simulink model "ControlModel"  (R2020b)
settings: Solver=VariableStepAuto  StartTime=0.0  StopTime=3  FixedStep=0.00001  RelTol=1e-3
InitFcn:
  | s = tf('s');
  | Telec = 1/10000000;
  | Tmech = Telec * 10;
  | CW = 1;
  | CCW = -1;
undefined symbols (not defined in the file or in its folder): DiscIntNeverNeededParam, lag, lead, magnitude, notch, rad
libraries: cstblocks x41, sharedtransform x7, simulink x6, aerolibutil x4, aerolibconvert2 x4, simulink_extras x3, sharedutil x1
(part 1 of 2)
settings Model: Creator=Iftah  LastModifiedBy=vguidance01

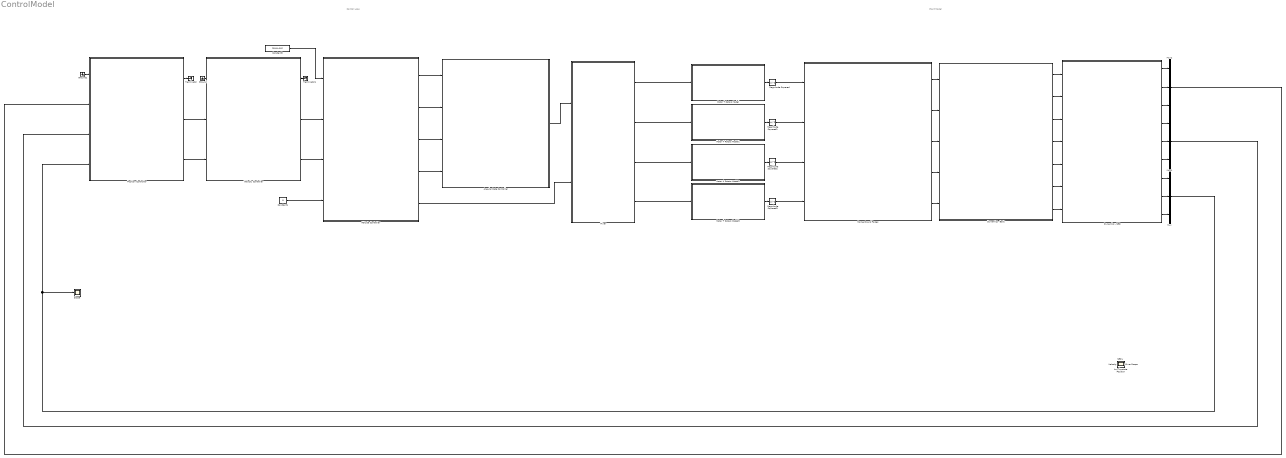
== system ControlModel ==
  note: Plant Model
  note: Control Loop
  Angular Rate Controller : Subsystem  mask{MC_ROLLRATE_K=1, MC_ROLLRATE_P=3, MC_ROLLRATE_I=0.8, MC_ROLLRATE_D=0.4, MC_RR_INT_LIM=101, MC_PITCHRATE_K=1, MC_PITCHRATE_P=3, MC_PITCHRATE_I=0.6, MC_PITCHRATE_D=0.4, MC_PR_INT_LIM=100, MC_YAWRATE_K=1, MC_YAWRATE_P=0.2, MC_YAWRATE_I=0.08, MC_YAWRATE_D=0.001, MC_YR_INT_LIM=100, IMU_DGYRO_CUTOFF=0, IMU_GYRO_CUTOFF=0}
      mask prompts: MC_ROLLRATE_K "MC_ROLLRATE_K ="; MC_ROLLRATE_P "MC_ROLLRATE_P ="; MC_ROLLRATE_I "MC_ROLLRATE_I ="; MC_ROLLRATE_D "MC_ROLLRATE_D ="; MC_RR_INT_LIM "MC_RR_INT_LIM ="; MC_PITCHRATE_K "MC_PITCHRATE_K ="; MC_PITCHRATE_P "MC_PITCHRATE_P ="; MC_PITCHRATE_I "MC_PITCHRATE_I ="; MC_PITCHRATE_D "MC_PITCHRATE_D ="; MC_PR_INT_LIM "MC_PR_INT_LIM ="; MC_YAWRATE_K "MC_YAWRATE_K ="; MC_YAWRATE_P "MC_YAWRATE_P ="; MC_YAWRATE_I "MC_YAWRATE_I ="; MC_YAWRATE_D "MC_YAWRATE_D ="; MC_YR_INT_LIM "MC_YR_INT_LIM ="; IMU_DGYRO_CUTOFF "IMU_DGYRO_CUTOFF ="; IMU_GYRO_CUTOFF "IMU_GYRO_CUTOFF ="
      mask DialogControl DescTextVar Prompt: Angular rate controller, based on PX4 architecture
      mask DialogControl ROLL Prompt: Roll
      mask DialogControl PITCH Prompt: Pitch
      mask DialogControl YAW Prompt: Yaw
      mask Display:
      | disp('Angular Rate Controller')
      | 
      | port_label('input',1,'d\phi_{cmd}','texmode','on')
      | port_label('input',2,'d\theta_{cmd}','texmode','on')
      | port_label('input',3,'d\psi_{cmd}','texmode','on')
      | port_label('input',4,'Gyro','texmode','on')
      | 
      | port_label('output',1,'\delta_{cmd}','texmode','on')
  Attitude Controller : Subsystem  mask{MC_ROLL_P=1, MC_ROLLRATE_MAX=0.5, MC_ACRO_R_MAX=10, MC_YAW_WEIGHT=0.1, m=1.37}
      mask prompts: MC_ROLL_P "MC_ROLL_P ="; MC_ROLLRATE_MAX "MC_ROLLRATE_MAX ="; MC_ACRO_R_MAX "MC_ACRO_R_MAX ="; MC_YAW_WEIGHT "MC_YAW_WEIGHT ="; m "m [kg] ="
      mask DialogControl DescTextVar Prompt: Attitude Controller - based on PX4 architecture
      mask Display:
      | disp('Attitude Controller')
      | 
      | port_label('input',1,'ACCEL. S.P')
      | port_label('input',3,'Accel')
      | port_label('input',2,'Gyro')
      | port_label('input',4,'\psi_{cmd}','texmode','on')
      | 
      | port_label('output',1,'d\phi_{cmd}','texmode','on')
      | port_label('output',2,'d\theta_{cmd}','texmode','on')
      | port_label('output',3,'d\psi_{cmd}','texmode','on')
      | port_label('output',4,'Gyro','texmode','on')
      | port_label('output',5,'Thrust_{cmd}','texmode','on')
  Constant1 : Constant  Value=0  SampleTime=Tmech
  Constant3 : Constant  Value=[10;0;-10]  SampleTime=Tmech
  Dynamics - Body : Subsystem  mask{Ixx=0.0115118, Iyy=0.0365651, Izz=0.0290742, Jr=2.8e-6, d=0.25}
      mask prompts: Ixx "Ixx [kg*m^2] ="; Iyy "Iyy [kg*m^2] ="; Izz "Izz [kg*m^2]="; Jr "Jl [kg*m^2]="; d "d [m] ="
      mask DialogControl DescTextVar Prompt: This model represents the body-frame dyanmics. Enter the MOIs of the system
      mask Display:
      | disp('Body Dyanmics','texmode','on')
      | 
      | port_label('input',1,'T','texmode','on')
      | port_label('input',2,'Roll Thrust','texmode','on')
      | port_label('input',3,'Pitch Thrust','texmode','on')
      | port_label('input',4,'Yaw Thrust','texmode','on')
      | port_label('input',5,'Angular Velocity','texmode','on')
      | 
      | port_label('output',2,'\phi','texmode','on')
      | port_label('output',3,'\theta','texmode','on')
      | port_label('output',4,'\psi','texmode','on')
      | port_label('output',1,'T','texmode','on')
      | port_label('output',5,'d\phi','texmode','on')
      | port_label('output',6,'d\theta','texmode','on')
      | port_label('output',7,'d\psi','texmode','on')
  Dynamics - NED : Subsystem  mask{g=9.81, m=1.37, Ax=0.007, Ay=0.007, Az=0.007}
      mask prompts: g "g [m/s^2] ="; m "m [kg] ="; Ax "Ax [kg/s] ="; Ay "Ay [kg/s]="; Az "Az [kg/s]="
      mask DialogControl DescTextVar Prompt: This block transform the body dyanmics to NED. Choose the mass, gravity, and Ax,Ay,Az - drag coeff.
      mask Display:
      | disp('NED Dyanmics','texmode','on')
      | 
      | port_label('input',2,'\phi','texmode','on')
      | port_label('input',3,'\theta','texmode','on')
      | port_label('input',4,'\psi','texmode','on')
      | port_label('input',1,'T','texmode','on')
      | port_label('input',5,'d\phi','texmode','on')
      | port_label('input',6,'d\theta','texmode','on')
      | port_label('input',7,'d\psi','texmode','on')
      | 
      | % port_label('output',1,'X','texmode','on')
      | % port_label('output',2,'Y','texmode','on')
      | % port_label('output',3,'Z','texmode','on')
      | 
      | % port_label('output',4,'dX','texmode','on')
      | % port_label('output',5,'dY','texmode','on')
      | % port_label('output',6,'dZ','texmode','on')
      | 
      | port_label('output',7,'ddx','texmode','on')
      | port_label('output',8,'ddy','texmode','on')
      | port_label('output',9,'ddz','texmode','on')
      | 
      | port_label('output',4,'d\phi','texmode','on')
      | port_label('output',5,'d\theta','texmode','on')
      | port_label('output',6,'d\psi','texmode','on')
      | 
      | port_label('output',1,'\phi','texmode','on')
      | port_label('output',2,'\theta','texmode','on')
      | port_label('output',3,'\psi','texmode','on')
  Ground : Ground
  Ground1 : Ground
  Magnitude Squared{,1..3} (4 alike) : Math  Operator=magnitude^2  SaturateOnIntegerOverflow=on
  Mixer : Subsystem  mask{Ct=5.947e-5, Cq=7.9217e-7, d=0.25}
      mask prompts: Ct "Ct ="; Cq "Cq ="; d "d [m] ="
      mask Display:
      | disp('Mixer')
      | 
      | port_label('input',1,'\delta_{cmd}','texmode','on')
      | port_label('input',2,'Thrust_{cmd}','texmode','on')
      | 
      | port_label('output',1,'\Omega_{1cmd}','texmode','on')
      | port_label('output',2,'\Omega_{2cmd}','texmode','on')
      | port_label('output',3,'\Omega_{3cmd}','texmode','on')
      | port_label('output',4,'\Omega_{4cmd}','texmode','on')
  Moments and Forces : Subsystem  mask{Ct=5.947e-5, Cq=7.9217e-7, d=0.25}
      mask prompts: Ct "Ct ="; Cq "Cq ="; d "d [m] ="
      mask DialogControl DescTextVar Prompt: This block represents the moment and force calculations. Supply the Ct - thrust constant and Cq is the drag consant. d is the quadrotor arm's length
      mask DialogControl Container3 Prompt: Constants:
      mask Display:
      | disp('Moments and Forces')
      | 
      | port_label('input',1,'\Omega_{1}^2','texmode','on')
      | port_label('input',2,'\Omega_{2}^2','texmode','on')
      | port_label('input',3,'\Omega_{3}^2','texmode','on')
      | port_label('input',4,'\Omega_{4}^2','texmode','on')
      | 
      | port_label('output',1,'T','texmode','on')
      | port_label('output',2,'Roll Thrust','texmode','on')
      | port_label('output',3,'Pitch Thrust','texmode','on')
      | port_label('output',4,'Yaw Thrust','texmode','on')
      | port_label('output',5,'Angular Velocity','texmode','on')
  Motor + Rotors Model : Subsystem  mask{R=0.127, L=1.6968e-4, Kt=1/104.7197, Kb=1/104.7197, Jm=3.38e-7, VSat=12.6, CurrentSat=30, Kk=1000, Kv=1, Jl=2.8e-6, Variance=0, Mean=0}
      mask prompts: R "R [Ohm] ="; L "L [H] ="; Kt "Kt [N*m/amp] ="; Kb "Kb [V/rad/sec] ="; Jm "Jm [kg*m^2] ="; VSat "Max. Voltage [V] ="; CurrentSat "Max. Current [A] ="; Kk "Kk ="; Kv "Kv ="; Jl "Jl ="; Variance "Noise Variance"; Mean "Noise Mean"
      mask DialogControl DescGroupVar Prompt: Brushless Motor - Prop  Model
      mask DialogControl DescTextVar Prompt: This block simulates the brushless motor - propeller dynamics, with no gear system. Choose the motor's elements and the propeller constants.
      mask DialogControl Container5 Prompt: Motor Parameters:
      mask DialogControl Container6 Prompt: Propeller Parameters:
      mask Display:
      | disp('Motor 1')
      | 
      | port_label('input',1,'\Omega_{1cmd}','texmode','on')
      | 
      | port_label('output',1,'\Omega_1','texmode','on')
  Motor + Rotors Model1 : Subsystem  mask{R=0.127, L=1.6968e-4, Kt=1/104.7197, Kb=1/104.7197, Jm=3.38e-7, VSat=12.6, CurrentSat=30, Kk=1000, Kv=1, Jl=2.8e-6, Variance=0, Mean=0}
      mask prompts: R "R [Ohm] ="; L "L [H] ="; Kt "Kt [N*m/amp] ="; Kb "Kb [V/rad/sec] ="; Jm "Jm [kg*m^2] ="; VSat "Max. Voltage [V] ="; CurrentSat "Max. Current [A] ="; Kk "Kk ="; Kv "Kv ="; Jl "Jl ="; Variance "Noise Variance"; Mean "Noise Mean"
      mask DialogControl DescGroupVar Prompt: Brushless Motor - Prop  Model
      mask DialogControl DescTextVar Prompt: This block simulates the brushless motor - propeller dynamics, with no gear system. Choose the motor's elements and the propeller constants.
      mask DialogControl Container5 Prompt: Motor Parameters:
      mask DialogControl Container6 Prompt: Propeller Parameters:
      mask Display:
      | disp('Motor 2')
      | 
      | port_label('input',1,'\Omega_{2cmd}','texmode','on')
      | 
      | port_label('output',1,'\Omega_2','texmode','on')
  Motor + Rotors Model2 : Subsystem  mask{R=0.127, L=1.6968e-4, Kt=1/104.7197, Kb=1/104.7197, Jm=3.38e-7, VSat=12.6, CurrentSat=30, Kk=1000, Kv=1, Jl=2.8e-6, Variance=0, Mean=0}
      mask prompts: R "R [Ohm] ="; L "L [H] ="; Kt "Kt [N*m/amp] ="; Kb "Kb [V/rad/sec] ="; Jm "Jm [kg*m^2] ="; VSat "Max. Voltage [V] ="; CurrentSat "Max. Current [A] ="; Kk "Kk ="; Kv "Kv ="; Jl "Jl ="; Variance "Noise Variance"; Mean "Noise Mean"
      mask DialogControl DescGroupVar Prompt: Brushless Motor - Prop  Model
      mask DialogControl DescTextVar Prompt: This block simulates the brushless motor - propeller dynamics, with no gear system. Choose the motor's elements and the propeller constants.
      mask DialogControl Container5 Prompt: Motor Parameters:
      mask DialogControl Container6 Prompt: Propeller Parameters:
      mask Display:
      | disp('Motor 3')
      | 
      | port_label('input',1,'\Omega_{3cmd}','texmode','on')
      | 
      | port_label('output',1,'\Omega_3','texmode','on')
  Motor + Rotors Model3 : Subsystem  mask{R=0.127, L=1.6968e-4, Kt=1/104.7197, Kb=1/104.7197, Jm=3.38e-7, VSat=12.6, CurrentSat=30, Kk=1000, Kv=1, Jl=2.8e-6, Variance=0, Mean=0}
      mask prompts: R "R [Ohm] ="; L "L [H] ="; Kt "Kt [N*m/amp] ="; Kb "Kb [V/rad/sec] ="; Jm "Jm [kg*m^2] ="; VSat "Max. Voltage [V] ="; CurrentSat "Max. Current [A] ="; Kk "Kk ="; Kv "Kv ="; Jl "Jl ="; Variance "Noise Variance"; Mean "Noise Mean"
      mask DialogControl DescGroupVar Prompt: Brushless Motor - Prop  Model
      mask DialogControl DescTextVar Prompt: This block simulates the brushless motor - propeller dynamics, with no gear system. Choose the motor's elements and the propeller constants.
      mask DialogControl Container5 Prompt: Motor Parameters:
      mask DialogControl Container6 Prompt: Propeller Parameters:
      mask Display:
      | disp('Motor 4')
      | 
      | port_label('input',1,'\Omega_{4cmd}','texmode','on')
      | 
      | port_label('output',1,'\Omega_4','texmode','on')
  Mux : Mux  Inputs=3
  Mux1 : Mux  Inputs=3
  Mux2 : Mux  Inputs=3
  Position Controller : Subsystem  mask{MPC_XY_P=1, MPC_XY_VEL_MAX=10, MPC_Z_P=1, MPC_Z_VEL_MAX_UP=100, MPC_Z_VEL_MAX_DOWN=-100}
      mask prompts: MPC_XY_P "MPC_XY_P ="; MPC_XY_VEL_MAX "MPC_XY_VEL_MAX ="; MPC_Z_P "MPC_Z_P ="; MPC_Z_VEL_MAX_UP "MPC_Z_VEL_MAX_UP ="; MPC_Z_VEL_MAX_DOWN "MPC_Z_VEL_MAX_DOWN ="
      mask DialogControl DescTextVar Prompt: Position Controller - based on PX4 architecture
      mask Display:
      | disp('Position Controller')
      | 
      | port_label('input',1,'POS. S.P')
      | port_label('input',4,'Accel')
      | port_label('input',3,'Gyro')
      | port_label('input',2,'Mag')
      | 
      | port_label('output',1,'VEL. S.P','texmode','on')
      | port_label('output',3,'Accel','texmode','on')
      | port_label('output',2,'Gyro','texmode','on')
  Scope : Scope
  Terminator : Terminator
  Terminator1 : Terminator
  Velocity Controller : Subsystem  mask{MPC_XY_VEL_P_ACC=1, MPC_XY_VEL_I_ACC=0.1, MPC_XY_VEL_D_ACC=0.05, MPC_Z_VEL_P_ACC=1, MPC_Z_VEL_I_ACC=0.1, MPC_Z_VEL_D_ACC=0.05, MPC_VELD_LP=0, MPC_TILTMAX_AIR=1000, MPC_THR_MAX=10000}
      mask prompts: MPC_XY_VEL_P_ACC "MPC_XY_VEL_P_ACC ="; MPC_XY_VEL_I_ACC "MPC_XY_VEL_I_ACC ="; MPC_XY_VEL_D_ACC "MPC_XY_VEL_D_ACC ="; MPC_Z_VEL_P_ACC "MPC_Z_VEL_P_ACC ="; MPC_Z_VEL_I_ACC "MPC_Z_VEL_I_ACC ="; MPC_Z_VEL_D_ACC "MPC_Z_VEL_D_ACC ="; MPC_VELD_LP "MPC_VELD_LP ="; MPC_TILTMAX_AIR "MPC_TILTMAX_AIR ="; MPC_THR_MAX "MPC_THR_MAX ="
      mask DialogControl DescTextVar Prompt: Velocity Controller - based on PX4 architecture
      mask DialogControl Container3 Prompt: XY -  Velocity
      mask DialogControl Container4 Prompt: Z - Velocity
      mask DialogControl Container5 Prompt: General Parameters
      mask Display:
      | disp('Velocity Controller')
      | 
      | port_label('input',1,'VEL. S.P')
      | port_label('input',3,'Accel')
      | port_label('input',2,'Gyro')
      | 
      | port_label('output',1,'ACCEL. S.P','texmode','on')
      | port_label('output',3,'Accel','texmode','on')
      | port_label('output',2,'Gyro','texmode','on')
  Angular Rate : Scope
  Body : Scope
  Forces : Scope
  Mixer Scope : Scope
  Motor 1 : Scope
  NED : Scope
  Position : Scope
  Thrust : Scope
  Velocity : Scope
  wires:
  Motor + Rotors Model1/1(Velocity_feedback) -> Magnitude Squared1/1
  Motor + Rotors Model/1(Velocity_feedback) -> Magnitude Squared/1
  Motor + Rotors Model3/1(Velocity_feedback) -> Magnitude Squared3/1
  Motor + Rotors Model2/1(Velocity_feedback) -> Magnitude Squared2/1
  Moments and Forces/5(Omega_R) -> Dynamics - Body/5(In5)
  Moments and Forces/4(Yaw) -> Dynamics - Body/4(In2)
  Moments and Forces/3(Pitch) -> Dynamics - Body/3(In4)
  Moments and Forces/2(Roll) -> Dynamics - Body/2(In3)
  Moments and Forces/1(Thrust) -> Dynamics - Body/1(In1)
  Dynamics - Body/4(Out3) -> Dynamics - NED/4(psi_in)
  Dynamics - Body/3(Out2) -> Dynamics - NED/3(theta_in)
  Dynamics - Body/2(Out1) -> Dynamics - NED/2(phi_in)
  Dynamics - Body/1(Out4) -> Dynamics - NED/1(T)
  Dynamics - Body/6(Out6) -> Dynamics - NED/6(dtheta_in)
  Dynamics - Body/5(Out5) -> Dynamics - NED/5(dphi_in)
  Dynamics - Body/7(Out7) -> Dynamics - NED/7(dpsi_in)
  Mixer/4(Omega 4) -> Motor + Rotors Model3/1(Velocity_cmd)
  Mixer/2(Omega 2) -> Motor + Rotors Model1/1(Velocity_cmd)
  Mixer/3(Omega 3) -> Motor + Rotors Model2/1(Velocity_cmd)
  Dynamics - NED/9(ddz) -> Mux/3
  Dynamics - NED/8(ddy) -> Mux/2
  Dynamics - NED/7(ddx) -> Mux/1
  Dynamics - NED/5(dtheta) -> Mux1/2
  Dynamics - NED/6(dpsi) -> Mux1/3
  Dynamics - NED/4(dphi) -> Mux1/1
  Dynamics - NED/3(psi) -> Mux2/3
  Dynamics - NED/2(theta) -> Mux2/2
  Dynamics - NED/1(phi) -> Mux2/1
  Position Controller/3(Accel.out) -> Velocity Controller/3(Accel)
  Position Controller/2(Gyro.out) -> Velocity Controller/2(Gyro)
  Mixer/1(Omega 1) -> Motor + Rotors Model/1(Velocity_cmd)
  Velocity Controller/2(Gyro.out) -> Attitude Controller/2(Gyro)
  Velocity Controller/3(Accel.out) -> Attitude Controller/3(Accel)
  Constant1/1 -> Attitude Controller/4(Yaw.SP)
  Attitude Controller/4(Outport) -> Angular Rate Controller/4(Gyro)
  Magnitude Squared3/1 -> Moments and Forces/4(In4)
  Magnitude Squared2/1 -> Moments and Forces/3(In3)
  Magnitude Squared1/1 -> Moments and Forces/2(In2)
  Magnitude Squared/1 -> Moments and Forces/1(In1)
  Angular Rate Controller/1(Delta S.P) -> Mixer/1(Tau_roll,pitch,yaw)
  Mux2/1 -> Position Controller/2(Mag)
  Mux1/1 -> Position Controller/3(Gyro)
  Mux/1 -> Position Controller/4(Accel), Scope/1
  Attitude Controller/5(Thrust) -> Mixer/2(Thrust)
  Attitude Controller/1(dPhi_cmd) -> Angular Rate Controller/1(dphi_sp)
  Attitude Controller/2(dTheta_cmd) -> Angular Rate Controller/2(dtheta_sp)
  Attitude Controller/3(dPsi_cmd) -> Angular Rate Controller/3(dpsi_sp)
  Position Controller/1(Vel S.P) -> Terminator/1
  Ground/1 -> Velocity Controller/1(Setpoints)
  Constant3/1 -> Attitude Controller/1(Setpoints)
  Ground1/1 -> Position Controller/1(Setpoints)
  Velocity Controller/1(Vel S.P) -> Terminator1/1

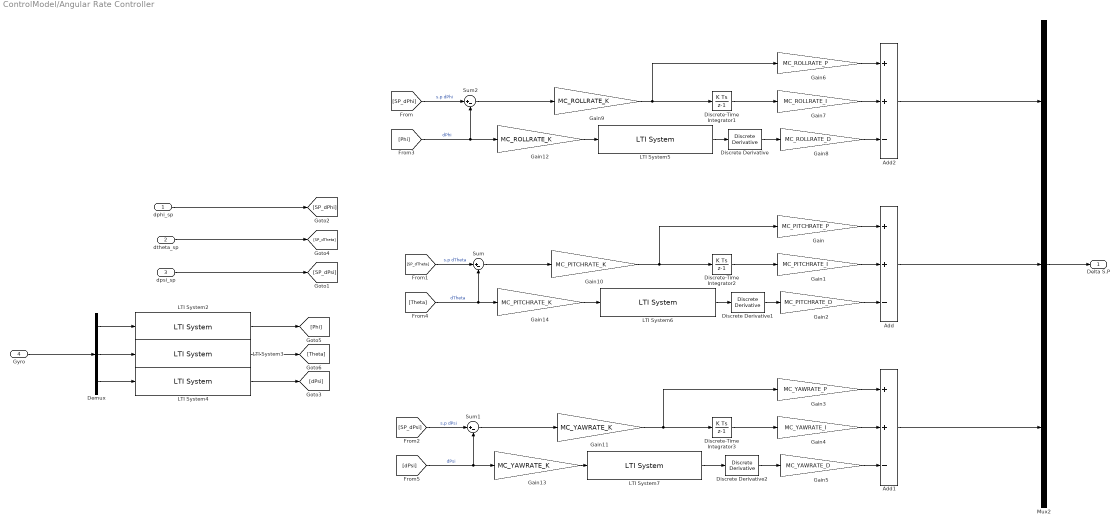
== system ControlModel/Angular Rate Controller ==
  dphi_sp : Inport
  dtheta_sp : Inport  Port=2
  dpsi_sp : Inport  Port=3
  Gyro : Inport  Port=4
  Add : Sum  Inputs=++-
  Add1 : Sum  Inputs=++-
  Add2 : Sum  Inputs=++-
  Demux : Demux  Outputs=3
  Discrete Derivative : simulink/Discrete/Discrete Derivative  gainval=1.0  ICPrevScaledInput=0.0  OutMin=[]  OutMax=[]  OutDataType=fixdt(1, 16)  OutScaling=2^-10  DoSatur=off
  Discrete Derivative1 : simulink/Discrete/Discrete Derivative  gainval=1.0  ICPrevScaledInput=0.0  OutMin=[]  OutMax=[]  OutDataType=fixdt(1, 16)  OutScaling=2^-10  DoSatur=off
  Discrete Derivative2 : simulink/Discrete/Discrete Derivative  gainval=1.0  ICPrevScaledInput=0.0  OutMin=[]  OutMax=[]  OutDataType=fixdt(1, 16)  OutScaling=2^-10  DoSatur=off
  Discrete-Time Integrator1 : DiscreteIntegrator  SampleTime=Tmech  LimitOutput=on  UpperSaturationLimit=MC_RR_INT_LIM  LowerSaturationLimit=-MC_RR_INT_LIM  ICPrevOutput=DiscIntNeverNeededParam  ICPrevScaledInput=DiscIntNeverNeededParam
  Discrete-Time Integrator2 : DiscreteIntegrator  SampleTime=Tmech  LimitOutput=on  UpperSaturationLimit=MC_PR_INT_LIM  LowerSaturationLimit=-MC_PR_INT_LIM  ICPrevOutput=DiscIntNeverNeededParam  ICPrevScaledInput=DiscIntNeverNeededParam
  Discrete-Time Integrator3 : DiscreteIntegrator  SampleTime=Tmech  LimitOutput=on  UpperSaturationLimit=MC_YR_INT_LIM  LowerSaturationLimit=-MC_YR_INT_LIM  ICPrevOutput=DiscIntNeverNeededParam  ICPrevScaledInput=DiscIntNeverNeededParam
  Gain : Gain  Gain=MC_PITCHRATE_P
  Gain1 : Gain  Gain=MC_PITCHRATE_I
  Gain10 : Gain  Gain=MC_PITCHRATE_K
  Gain11 : Gain  Gain=MC_YAWRATE_K
  Gain12 : Gain  Gain=MC_ROLLRATE_K
  Gain13 : Gain  Gain=MC_YAWRATE_K
  Gain14 : Gain  Gain=MC_PITCHRATE_K
  Gain2 : Gain  Gain=MC_PITCHRATE_D
  Gain3 : Gain  Gain=MC_YAWRATE_P
  Gain4 : Gain  Gain=MC_YAWRATE_I
  Gain5 : Gain  Gain=MC_YAWRATE_D
  Gain6 : Gain  Gain=MC_ROLLRATE_P
  Gain7 : Gain  Gain=MC_ROLLRATE_I
  Gain8 : Gain  Gain=MC_ROLLRATE_D
  Gain9 : Gain  Gain=MC_ROLLRATE_K
  LTI System2 : cstblocks/LTI System  sys=c2d(tf(1,[IMU_GYRO_CUTOFF 1]),Tmech)  IC=[]
  LTI System3 : cstblocks/LTI System  sys=c2d(tf(1,[IMU_GYRO_CUTOFF 1]),Tmech)  IC=[]
  LTI System4 : cstblocks/LTI System  sys=c2d(tf(1,[IMU_GYRO_CUTOFF 1]),Tmech)  IC=[]
  LTI System5 : cstblocks/LTI System  sys=c2d(tf(1,[IMU_DGYRO_CUTOFF 1]),Tmech)  IC=[]
  LTI System6 : cstblocks/LTI System  sys=c2d(tf(1,[IMU_DGYRO_CUTOFF 1]),Tmech)  IC=[]
  LTI System7 : cstblocks/LTI System  sys=c2d(tf(1,[IMU_DGYRO_CUTOFF 1]),Tmech)  IC=[]
  Mux2 : Mux  Inputs=3
  Sum : Sum  Inputs=|+-
  Sum1 : Sum  Inputs=|+-
  Sum2 : Sum  Inputs=|+-
  Delta S.P : Outport
  wires:
  dtheta_sp/1 -> [SP_dTheta]
  LTI System6/1 -> Discrete Derivative1/1
  Sum/1 -> Gain10/1
  Discrete-Time Integrator2/1 -> Gain1/1
  Gain2/1 -> Add/3
  Gain1/1 -> Add/2
  Gain/1 -> Add/1
  Gain3/1 -> Add1/1
  Gain4/1 -> Add1/2
  Gain5/1 -> Add1/3
  Discrete-Time Integrator3/1 -> Gain4/1
  Sum1/1 -> Gain11/1
  LTI System7/1 -> Discrete Derivative2/1
  [dPsi] -> Gain13/1, Sum1/2  "dPsi"
  [SP_dPsi] -> Sum1/1  "s.p dPsi"
  Add/1 -> Mux2/2
  Mux2/1 -> Delta S.P/1
  Gain6/1 -> Add2/1
  Gain7/1 -> Add2/2
  Gain8/1 -> Add2/3
  Discrete-Time Integrator1/1 -> Gain7/1
  Sum2/1 -> Gain9/1
  LTI System5/1 -> Discrete Derivative/1
  [SP_dPhi] -> Sum2/1  "s.p dPhi"
  [SP_dTheta] -> Sum/1  "s.p dTheta"
  [Phi] -> Gain12/1, Sum2/2  "dPhi"
  [Theta] -> Gain14/1, Sum/2  "dTheta"
  Add2/1 -> Mux2/1
  Add1/1 -> Mux2/3
  Discrete Derivative/1 -> Gain8/1
  Discrete Derivative1/1 -> Gain2/1
  Discrete Derivative2/1 -> Gain5/1
  Gain9/1 -> Discrete-Time Integrator1/1, Gain6/1
  Gain10/1 -> Discrete-Time Integrator2/1, Gain/1
  Gain11/1 -> Discrete-Time Integrator3/1, Gain3/1
  Gain12/1 -> LTI System5/1
  Gain13/1 -> LTI System7/1
  Gain14/1 -> LTI System6/1
  Gyro/1 -> Demux/1
  Demux/1 -> LTI System2/1
  Demux/2 -> LTI System3/1
  Demux/3 -> LTI System4/1
  LTI System2/1 -> [Phi]
  LTI System3/1 -> [Theta]
  LTI System4/1 -> [dPsi]
  dpsi_sp/1 -> [SP_dPsi]
  dphi_sp/1 -> [SP_dPhi]

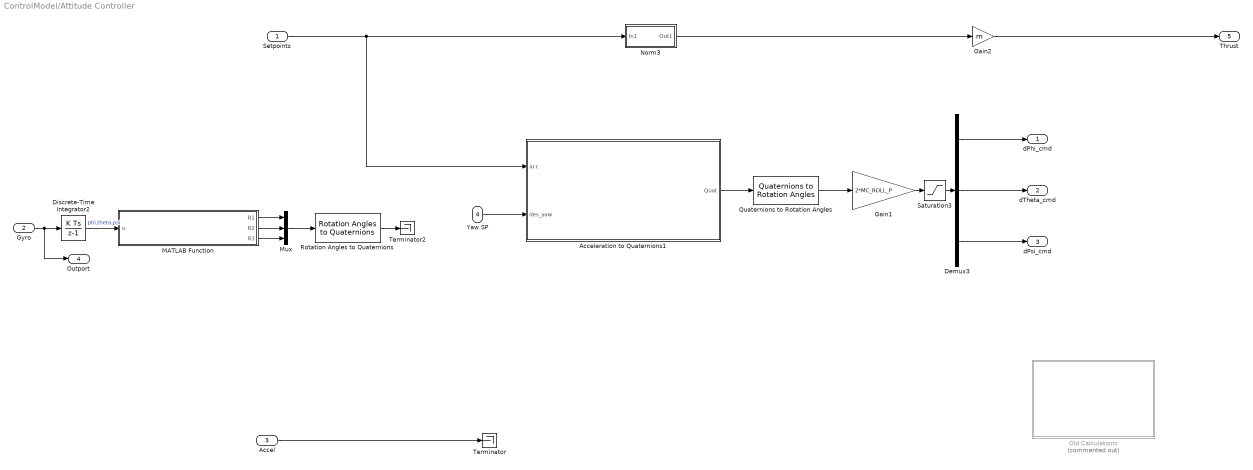
== system ControlModel/Attitude Controller ==
  Setpoints : Inport
  Gyro : Inport  Port=2
  Accel : Inport  Port=3
  Yaw.SP : Inport  Port=4
  Acceleration to Quaternions1 : Subsystem
      mask Display:
      | disp('Acceleration2Quaternions')
      | 
      | port_label('input',1,'Acc_{cmd}','texmode','on')
      | port_label('input',2,'Yaw_{cmd}','texmode','on')
      | 
      | 
      | port_label('output',1,'quat_{cmd}','texmode','on')
  Demux3 : Demux  Outputs=3
  Discrete-Time Integrator2 : DiscreteIntegrator  InitialCondition=[0.001;0.001;0.001]  SampleTime=-1  ICPrevOutput=DiscIntNeverNeededParam  ICPrevScaledInput=DiscIntNeverNeededParam
  Gain1 : Gain  Gain=2*MC_ROLL_P
  Gain2 : Gain  Gain=m
  MATLAB Function : MATLAB Function  TreatAsAtomicUnit=on
  Mux : Mux  Inputs=3
  Norm3 : Subsystem
      mask Display: disp('Norm')
  Old Calculations : Subsystem  Commented=on
  Quaternions to Rotation Angles : sharedtransform/Quaternions to Rotation Angles  rotationOrder=ZYX  aMode=aMode
      settings: SourceProductBaseCode=AE,PW,MT,UV,VE,VP
  Rotation Angles to Quaternions : sharedtransform/Rotation Angles to Quaternions  rotationOrder=ZYX  aMode=aMode
      settings: SourceProductBaseCode=AE,PW,MT,UV,VE,VP
  Saturation3 : Saturate  UpperLimit=MC_ROLLRATE_MAX  LowerLimit=-MC_ROLLRATE_MAX
  Terminator : Terminator
  Terminator2 : Terminator
  dPhi_cmd : Outport
  dTheta_cmd : Outport  Port=2
  dPsi_cmd : Outport  Port=3
  Outport : Outport  Port=4
  Thrust : Outport  Port=5
  wires:
  Discrete-Time Integrator2/1 -> MATLAB Function/1(u)  "phi,theta,psi"
  Gyro/1 -> Outport/1, Discrete-Time Integrator2/1
  Norm3/1(Out1) -> Gain2/1
  Accel/1 -> Terminator/1
  Setpoints/1 -> Acceleration to Quaternions1/1(acc), Norm3/1(In1)
  Gain1/1 -> Saturation3/1
  Saturation3/1 -> Demux3/1
  Gain2/1 -> Thrust/1
  Acceleration to Quaternions1/1(Quat) -> Quaternions to Rotation Angles/1
  Yaw.SP/1 -> Acceleration to Quaternions1/2(des_yaw)
  Rotation Angles to Quaternions/1 -> Terminator2/1
  MATLAB Function/2(R2) -> Mux/2
  MATLAB Function/1(R1) -> Mux/1
  MATLAB Function/3(R3) -> Mux/3
  Mux/1 -> Rotation Angles to Quaternions/1
  Quaternions to Rotation Angles/1 -> Gain1/1
  Demux3/1 -> dPhi_cmd/1
  Demux3/2 -> dTheta_cmd/1
  Demux3/3 -> dPsi_cmd/1

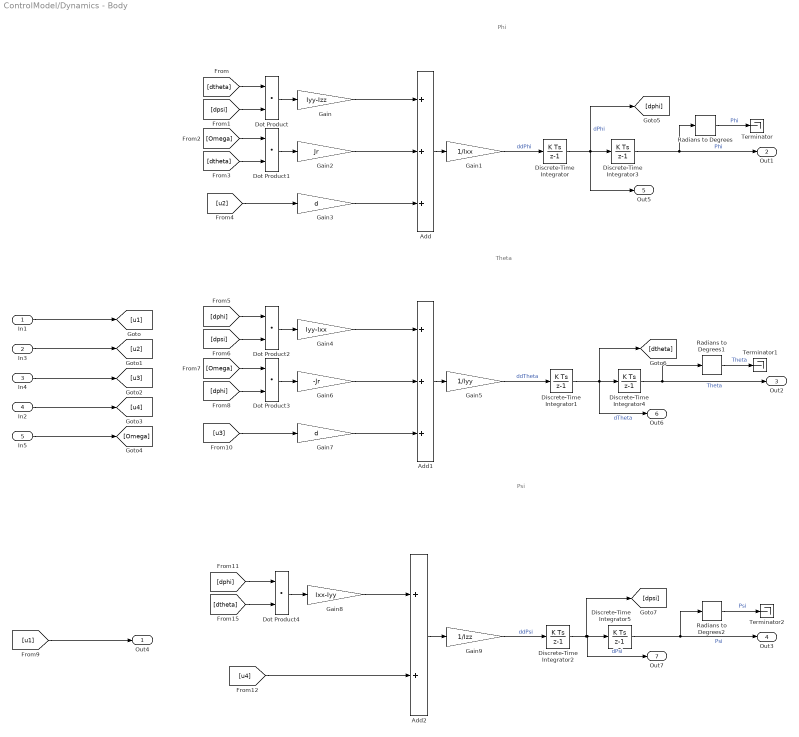
== system ControlModel/Dynamics - Body ==
  note: Phi
  note: Theta
  note: Psi
  In1 : Inport
  In3 : Inport  Port=2
  In4 : Inport  Port=3
  In2 : Inport  Port=4
  In5 : Inport  Port=5
  Add : Sum  Inputs=3
  Add1 : Sum  Inputs=3
  Add2 : Sum  Inputs=2
  Discrete-Time Integrator{,1..2,5} (4 alike) : DiscreteIntegrator  SampleTime=Tmech  ICPrevOutput=DiscIntNeverNeededParam  ICPrevScaledInput=DiscIntNeverNeededParam
  Discrete-Time Integrator3 : DiscreteIntegrator  SampleTime=Tmech  LimitOutput=on  UpperSaturationLimit=pi/2-0.001  LowerSaturationLimit=-pi/2+0.001  ICPrevOutput=DiscIntNeverNeededParam  ICPrevScaledInput=DiscIntNeverNeededParam
  Discrete-Time Integrator4 : DiscreteIntegrator  SampleTime=Tmech  LimitOutput=on  UpperSaturationLimit=pi/2 - 0.01  LowerSaturationLimit=-pi/2+0.01  ICPrevOutput=DiscIntNeverNeededParam  ICPrevScaledInput=DiscIntNeverNeededParam
  Dot Product{,1..4} (5 alike) : DotProduct  InputSameDT=on  OutDataTypeStr=Inherit: Inherit via internal rule
  Gain : Gain  Gain=Iyy-Izz
  Gain1 : Gain  Gain=1/Ixx
  Gain2 : Gain  Gain=Jr
  Gain3 : Gain  Gain=d
  Gain4 : Gain  Gain=Iyy-Ixx
  Gain5 : Gain  Gain=1/Iyy
  Gain6 : Gain  Gain=-Jr
  Gain7 : Gain  Gain=d
  Gain8 : Gain  Gain=Ixx-Iyy
  Gain9 : Gain  Gain=1/Izz
  Radians to Degrees : simulink_extras/Transformations/Radians to Degrees
  Radians to Degrees1 : simulink_extras/Transformations/Radians to Degrees
  Radians to Degrees2 : simulink_extras/Transformations/Radians to Degrees
  Terminator : Terminator
  Terminator1 : Terminator
  Terminator2 : Terminator
  Out4 : Outport
  Out1 : Outport  Port=2
  Out2 : Outport  Port=3
  Out3 : Outport  Port=4
  Out5 : Outport  Port=5
  Out6 : Outport  Port=6
  Out7 : Outport  Port=7
  wires:
  In1/1 -> [u1]
  In3/1 -> [u2]
  In4/1 -> [u3]
  In2/1 -> [u4]
  In5/1 -> [Omega]
  Discrete-Time Integrator/1 -> Discrete-Time Integrator3/1, Out5/1, [dphi]  "dPhi"
  Discrete-Time Integrator1/1 -> Out6/1, Discrete-Time Integrator4/1, [dtheta]  "dTheta"
  Discrete-Time Integrator2/1 -> [dpsi], Discrete-Time Integrator5/1, Out7/1  "dPsi"
  Discrete-Time Integrator3/1 -> Radians to Degrees/1, Out1/1  "Phi"
  Discrete-Time Integrator4/1 -> Radians to Degrees1/1, Out2/1  "Theta"
  Discrete-Time Integrator5/1 -> Radians to Degrees2/1, Out3/1  "Psi"
  [dpsi] -> Dot Product/2
  [dtheta] -> Dot Product/1
  Dot Product/1 -> Gain/1
  Gain/1 -> Add/1
  Gain1/1 -> Discrete-Time Integrator/1  "ddPhi"
  Add/1 -> Gain1/1
  [Omega] -> Dot Product1/1
  Dot Product1/1 -> Gain2/1
  [dtheta] -> Dot Product1/2
  Gain2/1 -> Add/2
  [u2] -> Gain3/1
  Gain7/1 -> Add1/3
  [u3] -> Gain7/1
  Gain6/1 -> Add1/2
  [dphi] -> Dot Product3/2
  Dot Product3/1 -> Gain6/1
  [Omega] -> Dot Product3/1
  Add1/1 -> Gain5/1
  Gain4/1 -> Add1/1
  Dot Product2/1 -> Gain4/1
  [dphi] -> Dot Product2/1
  [dpsi] -> Dot Product2/2
  Gain5/1 -> Discrete-Time Integrator1/1  "ddTheta"
  [dtheta] -> Dot Product4/2
  Dot Product4/1 -> Gain8/1
  Gain8/1 -> Add2/1
  Add2/1 -> Gain9/1
  Gain9/1 -> Discrete-Time Integrator2/1  "ddPsi"
  [dphi] -> Dot Product4/1
  [u4] -> Add2/2
  [u1] -> Out4/1
  Gain3/1 -> Add/3
  Radians to Degrees/1 -> Terminator/1  "Phi"
  Radians to Degrees1/1 -> Terminator1/1  "Theta"
  Radians to Degrees2/1 -> Terminator2/1  "Psi"

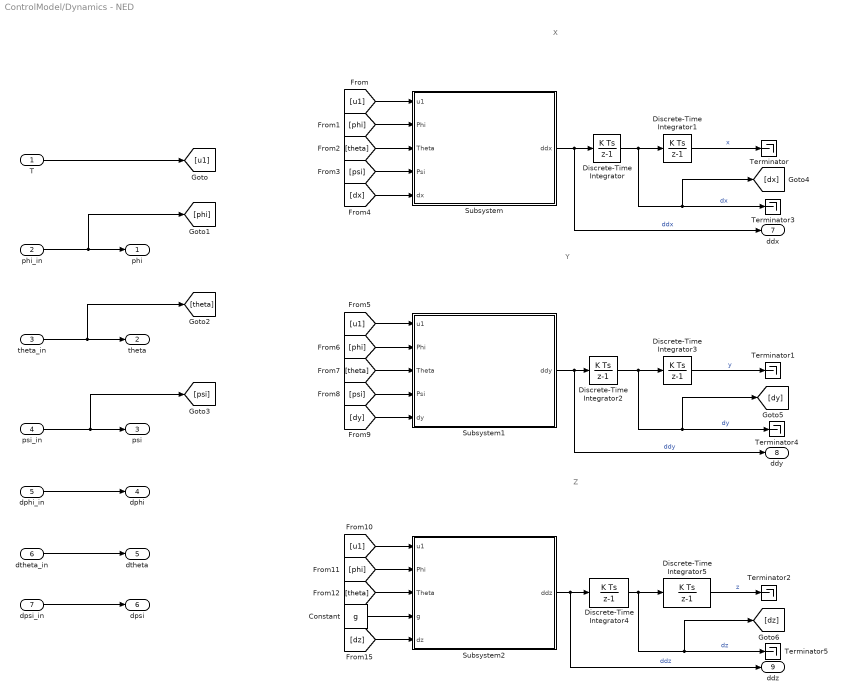
== system ControlModel/Dynamics - NED ==
  note: X
  note: Y
  note: Z
  T : Inport
  phi_in : Inport  Port=2
  theta_in : Inport  Port=3
  psi_in : Inport  Port=4
  dphi_in : Inport  Port=5
  dtheta_in : Inport  Port=6
  dpsi_in : Inport  Port=7
  Constant : Constant  Value=g  SampleTime=Tmech
  Discrete-Time Integrator{,1..3} (4 alike) : DiscreteIntegrator  SampleTime=Tmech  ICPrevOutput=DiscIntNeverNeededParam  ICPrevScaledInput=DiscIntNeverNeededParam
  Discrete-Time Integrator4 : DiscreteIntegrator  SampleTime=Tmech  LimitOutput=on  UpperSaturationLimit=0  ICPrevOutput=DiscIntNeverNeededParam  ICPrevScaledInput=DiscIntNeverNeededParam
  Discrete-Time Integrator5 : DiscreteIntegrator  SampleTime=Tmech  LimitOutput=on  UpperSaturationLimit=0  ICPrevOutput=DiscIntNeverNeededParam  ICPrevScaledInput=DiscIntNeverNeededParam
  Subsystem : Subsystem
  Subsystem1 : Subsystem
  Subsystem2 : Subsystem
  Terminator{,1..5} (6 alike) : Terminator
  phi : Outport
  theta : Outport  Port=2
  psi : Outport  Port=3
  dphi : Outport  Port=4
  dtheta : Outport  Port=5
  dpsi : Outport  Port=6
  ddx : Outport  Port=7
  ddy : Outport  Port=8
  ddz : Outport  Port=9
  wires:
  dpsi_in/1 -> dpsi/1
  dtheta_in/1 -> dtheta/1
  dphi_in/1 -> dphi/1
  psi_in/1 -> [psi], psi/1
  theta_in/1 -> [theta], theta/1
  phi_in/1 -> [phi], phi/1
  T/1 -> [u1]
  Discrete-Time Integrator1/1 -> Terminator/1  "x"
  Discrete-Time Integrator/1 -> Discrete-Time Integrator1/1, Terminator3/1, [dx]  "dx"
  Subsystem/1(ddx) -> Discrete-Time Integrator/1, ddx/1  "ddx"
  [u1] -> Subsystem/1(u1)
  [phi] -> Subsystem/2(Phi)
  [theta] -> Subsystem/3(Theta)
  [psi] -> Subsystem/4(Psi)
  [dx] -> Subsystem/5(dx)
  [dy] -> Subsystem1/5(dy)
  [psi] -> Subsystem1/4(Psi)
  [theta] -> Subsystem1/3(Theta)
  [phi] -> Subsystem1/2(Phi)
  [u1] -> Subsystem1/1(u1)
  Subsystem1/1(ddy) -> Discrete-Time Integrator2/1, ddy/1  "ddy"
  Discrete-Time Integrator2/1 -> Discrete-Time Integrator3/1, Terminator4/1, [dy]  "dy"
  Discrete-Time Integrator3/1 -> Terminator1/1  "y"
  Discrete-Time Integrator4/1 -> Discrete-Time Integrator5/1, [dz], Terminator5/1  "dz"
  Subsystem2/1(ddz) -> Discrete-Time Integrator4/1, ddz/1  "ddz"
  [u1] -> Subsystem2/1(u1)
  [phi] -> Subsystem2/2(Phi)
  [theta] -> Subsystem2/3(Theta)
  [dz] -> Subsystem2/5(dz)
  Discrete-Time Integrator5/1 -> Terminator2/1  "z"
  Constant/1 -> Subsystem2/4(g)

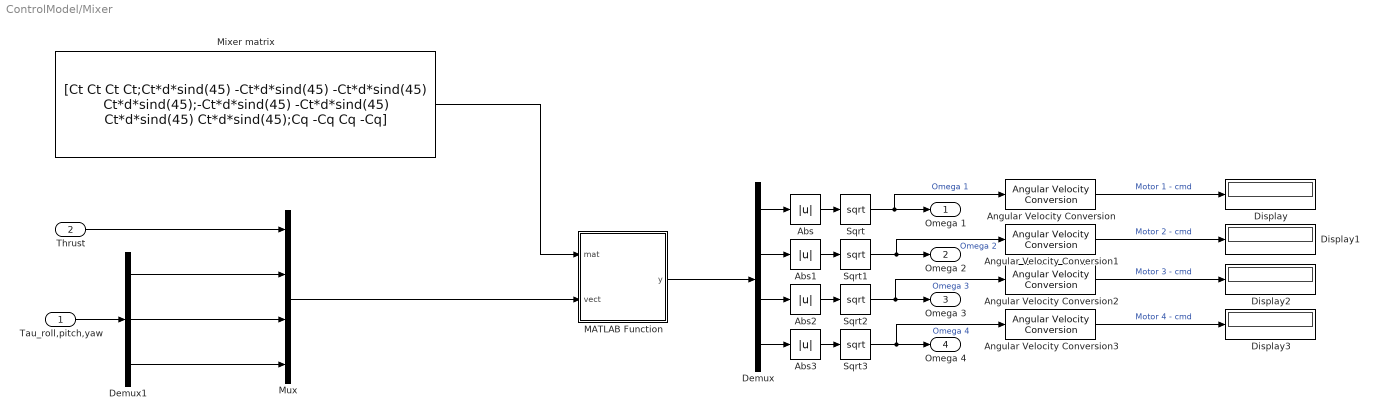
== system ControlModel/Mixer ==
  Tau_roll,pitch,yaw : Inport
  Thrust : Inport  Port=2
  Abs{,1..3} (4 alike) : Abs
  Angular Velocity Conversion{,1..3} (4 alike) : aerolibconvert2/Angular Velocity Conversion  IU=rad/s  OU=rpm
  Demux : Demux
  Demux1 : Demux  Outputs=3
  Display{,1..3} (4 alike) : Display
  MATLAB Function : MATLAB Function  TreatAsAtomicUnit=on
  Mixer matrix : Constant  StartFcn=|  Value=[Ct Ct Ct Ct;Ct*d*sind(45) -Ct*d*sind(45) -Ct*d*sind(45) Ct*d*sind(45);-Ct*d*sind(45) -Ct*d*sind(45) Ct*d*sind(45) Ct*d*sind(45);Cq -Cq Cq -Cq]  OutDataTypeStr=Inherit: Inherit via back propagation  SampleTime=Tmech
      | %p = Simulink.Mask.get('ControlsModels/Moments and Forces');
      | 
      | Ct = 0.025
      | Cq = 2e-6;
      | 
      | %Ct = p.getParameter('Ct');
      | %Cq =p.getParameter('Cq');
      | 
      | %Ct = str2double(Ct.Value);
      | %Cq = str2double(Cq.Value);
  Mux : Mux
  Sqrt{,1..3} (4 alike) : Sqrt  SaturateOnIntegerOverflow=on
  Omega 1 : Outport
  Omega 2 : Outport  Port=2
  Omega 3 : Outport  Port=3
  Omega 4 : Outport  Port=4
  wires:
  Thrust/1 -> Mux/1
  Demux/1 -> Abs/1
  Demux/2 -> Abs1/1
  Demux/3 -> Abs2/1
  Demux/4 -> Abs3/1
  MATLAB Function/1(y) -> Demux/1
  Mux/1 -> MATLAB Function/2(vect)
  Mixer matrix/1 -> MATLAB Function/1(mat)
  Sqrt/1 -> Angular Velocity Conversion/1, Omega 1/1  "Omega 1"
  Sqrt1/1 -> Angular Velocity Conversion1/1, Omega 2/1  "Omega 2"
  Sqrt2/1 -> Angular Velocity Conversion2/1, Omega 3/1  "Omega 3"
  Sqrt3/1 -> Angular Velocity Conversion3/1, Omega 4/1  "Omega 4"
  Tau_roll,pitch,yaw/1 -> Demux1/1
  Demux1/3 -> Mux/4
  Demux1/1 -> Mux/2
  Demux1/2 -> Mux/3
  Angular Velocity Conversion/1 -> Display/1  "Motor 1 - cmd"
  Angular Velocity Conversion1/1 -> Display1/1  "Motor 2 - cmd"
  Angular Velocity Conversion2/1 -> Display2/1  "Motor 3 - cmd"
  Angular Velocity Conversion3/1 -> Display3/1  "Motor 4 - cmd"
  Abs/1 -> Sqrt/1
  Abs1/1 -> Sqrt1/1
  Abs2/1 -> Sqrt2/1
  Abs3/1 -> Sqrt3/1

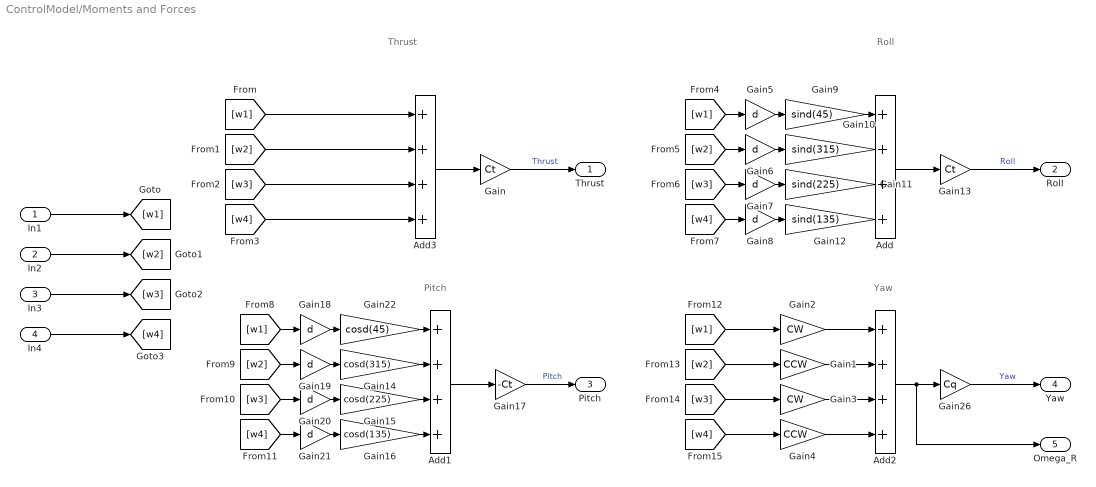
== system ControlModel/Moments and Forces ==
  note: Thrust
  note: Roll
  note: Pitch
  note: Yaw
  In1 : Inport
  In2 : Inport  Port=2
  In3 : Inport  Port=3
  In4 : Inport  Port=4
  Add{,1..3} (4 alike) : Sum  Inputs=4
  Gain : Gain  Gain=Ct
  Gain1 : Gain  Gain=CCW
  Gain10 : Gain  Gain=sind(315)
  Gain11 : Gain  Gain=sind(225)
  Gain12 : Gain  Gain=sind(135)
  Gain13 : Gain  Gain=Ct
  Gain14 : Gain  Gain=cosd(315)
  Gain15 : Gain  Gain=cosd(225)
  Gain16 : Gain  Gain=cosd(135)
  Gain17 : Gain  Gain=-Ct
  Gain{5..8,18..21} (8 alike) : Gain  Gain=d
  Gain2 : Gain  Gain=CW
  Gain22 : Gain  Gain=cosd(45)
  Gain26 : Gain  Gain=Cq
  Gain3 : Gain  Gain=CW
  Gain4 : Gain  Gain=CCW
  Gain9 : Gain  Gain=sind(45)
  Thrust : Outport
  Roll : Outport  Port=2
  Pitch : Outport  Port=3
  Yaw : Outport  Port=4
  Omega_R : Outport  Port=5
  wires:
  In1/1 -> [w1]
  In2/1 -> [w2]
  In3/1 -> [w3]
  In4/1 -> [w4]
  [w1] -> Add3/1
  [w2] -> Add3/2
  [w3] -> Add3/3
  [w4] -> Add3/4
  Gain/1 -> Thrust/1  "Thrust"
  [w4] -> Gain8/1
  [w3] -> Gain7/1
  [w2] -> Gain6/1
  [w1] -> Gain5/1
  Gain5/1 -> Gain9/1
  Gain6/1 -> Gain10/1
  Gain9/1 -> Add/1
  Gain10/1 -> Add/2
  Gain11/1 -> Add/3
  Gain7/1 -> Gain11/1
  Gain12/1 -> Add/4
  Gain8/1 -> Gain12/1
  Add/1 -> Gain13/1
  Gain13/1 -> Roll/1  "Roll"
  Gain17/1 -> Pitch/1  "Pitch"
  Add1/1 -> Gain17/1
  Gain21/1 -> Gain16/1
  Gain16/1 -> Add1/4
  Gain20/1 -> Gain15/1
  Gain15/1 -> Add1/3
  Gain14/1 -> Add1/2
  Gain22/1 -> Add1/1
  Gain19/1 -> Gain14/1
  Gain18/1 -> Gain22/1
  [w1] -> Gain18/1
  [w2] -> Gain19/1
  [w3] -> Gain20/1
  [w4] -> Gain21/1
  Gain26/1 -> Yaw/1  "Yaw"
  Add2/1 -> Omega_R/1, Gain26/1
  Gain4/1 -> Add2/4
  Gain3/1 -> Add2/3
  Gain1/1 -> Add2/2
  Gain2/1 -> Add2/1
  [w1] -> Gain2/1
  [w2] -> Gain1/1
  [w3] -> Gain3/1
  [w4] -> Gain4/1
  Add3/1 -> Gain/1

== system ControlModel/Motor + Rotors Model ==
  Velocity_cmd : Inport
  Add : Sum
  Current Controller : Subsystem
  Plant : Subsystem
  Random Number : RandomNumber  Mean=Mean  Variance=Variance  SampleTime=Tmech
  Rate Transition : RateTransition  OutPortSampleTime=Telec
  Rate Transition2 : RateTransition  OutPortSampleTime=Tmech
  Rate Transition3 : RateTransition  OutPortSampleTime=Telec
  Rate Transition4 : RateTransition  OutPortSampleTime=Tmech
  Saturation : Saturate  UpperLimit=VSat  LowerLimit=-VSat
  Saturation2 : Saturate  UpperLimit=CurrentSat  LowerLimit=-CurrentSat
  Sum : Sum  Inputs=-+|
  Sum1 : Sum  Inputs=|+-
  Velocity Controller : Subsystem
  Velocity_feedback : Outport
  wires:
  Plant/2(omega) -> Add/1
  Plant/1(Im) -> Rate Transition/1
  Rate Transition/1 -> Sum/1  "Current Feedback"
  Saturation/1 -> Plant/1(V_cmd)
  Sum/1 -> Current Controller/1(Current_error)
  Velocity Controller/1(Current_cmd) -> Rate Transition3/1
  Rate Transition3/1 -> Saturation2/1  "Current Command"
  Rate Transition2/1 -> Sum1/2, Velocity_feedback/1  "Velocity Feedback"
  Current Controller/1(Voltage_cmd) -> Saturation/1
  Add/1 -> Rate Transition2/1
  Random Number/1 -> Add/2
  Velocity_cmd/1 -> Rate Transition4/1
  Sum1/1 -> Velocity Controller/1(Velocity_error)
  Rate Transition4/1 -> Sum1/1  "Velocity Command"
  Saturation2/1 -> Sum/2

== system ControlModel/Motor + Rotors Model1 ==
  Velocity_cmd : Inport
  Add : Sum
  Current Controller : Subsystem
  Random Number : RandomNumber  Mean=Mean  Variance=Variance  SampleTime=Tmech
  Rate Transition : RateTransition  OutPortSampleTime=Telec
  Rate Transition1 : RateTransition  OutPortSampleTime=Tmech
  Rate Transition2 : RateTransition  OutPortSampleTime=Tmech
  Rate Transition3 : RateTransition  OutPortSampleTime=Telec
  Saturation : Saturate  UpperLimit=VSat  LowerLimit=-VSat
  Saturation2 : Saturate  UpperLimit=CurrentSat  LowerLimit=-CurrentSat
  Subsystem4 : Subsystem
  Sum : Sum  Inputs=-+|
  Sum1 : Sum  Inputs=|+-
  Velocity Controller : Subsystem
  Velocity_feedback : Outport
  wires:
  Random Number/1 -> Add/2
  Add/1 -> Rate Transition2/1
  Sum1/1 -> Velocity Controller/1(Velocity_error)
  Current Controller/1(Voltage_cmd) -> Saturation/1
  Rate Transition2/1 -> Velocity_feedback/1, Sum1/2
  Rate Transition3/1 -> Saturation2/1
  Velocity_cmd/1 -> Rate Transition1/1
  Velocity Controller/1(Current_cmd) -> Rate Transition3/1
  Sum/1 -> Current Controller/1(Current_error)
  Saturation/1 -> Subsystem4/1(V_cmd)
  Rate Transition/1 -> Sum/1
  Subsystem4/1(Im) -> Rate Transition/1
  Subsystem4/2(omega) -> Add/1
  Rate Transition1/1 -> Sum1/1
  Saturation2/1 -> Sum/2

== system ControlModel/Motor + Rotors Model2 ==
  Velocity_cmd : Inport
  Add : Sum
  Current Controller : Subsystem
  Random Number : RandomNumber  Mean=Mean  Variance=Variance  SampleTime=Tmech
  Rate Transition : RateTransition  OutPortSampleTime=Telec
  Rate Transition1 : RateTransition  OutPortSampleTime=Tmech
  Rate Transition2 : RateTransition  OutPortSampleTime=Tmech
  Rate Transition3 : RateTransition  OutPortSampleTime=Telec
  Saturation : Saturate  UpperLimit=VSat  LowerLimit=-VSat
  Saturation2 : Saturate  UpperLimit=CurrentSat  LowerLimit=-CurrentSat
  Subsystem4 : Subsystem
  Sum : Sum  Inputs=-+|
  Sum1 : Sum  Inputs=|+-
  Velocity Controller : Subsystem
  Velocity_feedback : Outport
  wires:
  Subsystem4/2(omega) -> Add/1
  Subsystem4/1(Im) -> Rate Transition/1
  Rate Transition/1 -> Sum/1
  Saturation/1 -> Subsystem4/1(V_cmd)
  Sum/1 -> Current Controller/1(Current_error)
  Velocity Controller/1(Current_cmd) -> Rate Transition3/1
  Velocity_cmd/1 -> Rate Transition1/1
  Rate Transition3/1 -> Saturation2/1
  Rate Transition2/1 -> Sum1/2, Velocity_feedback/1
  Current Controller/1(Voltage_cmd) -> Saturation/1
  Sum1/1 -> Velocity Controller/1(Velocity_error)
  Add/1 -> Rate Transition2/1
  Random Number/1 -> Add/2
  Rate Transition1/1 -> Sum1/1
  Saturation2/1 -> Sum/2

== system ControlModel/Motor + Rotors Model3 ==
  Velocity_cmd : Inport
  Add : Sum
  Current Controller : Subsystem
  Random Number : RandomNumber  Mean=Mean  Variance=Variance  SampleTime=Tmech
  Rate Transition : RateTransition  OutPortSampleTime=Telec
  Rate Transition1 : RateTransition  OutPortSampleTime=Tmech
  Rate Transition2 : RateTransition  OutPortSampleTime=Tmech
  Rate Transition3 : RateTransition  OutPortSampleTime=Telec
  Saturation : Saturate  UpperLimit=VSat  LowerLimit=-VSat
  Saturation2 : Saturate  UpperLimit=CurrentSat  LowerLimit=-CurrentSat
  Subsystem4 : Subsystem
  Sum : Sum  Inputs=-+|
  Sum1 : Sum  Inputs=|+-
  Velocity Controller : Subsystem
  Velocity_feedback : Outport
  wires:
  Random Number/1 -> Add/2
  Add/1 -> Rate Transition2/1
  Sum1/1 -> Velocity Controller/1(Velocity_error)
  Current Controller/1(Voltage_cmd) -> Saturation/1
  Rate Transition2/1 -> Velocity_feedback/1, Sum1/2
  Rate Transition3/1 -> Saturation2/1
  Velocity_cmd/1 -> Rate Transition1/1
  Velocity Controller/1(Current_cmd) -> Rate Transition3/1
  Sum/1 -> Current Controller/1(Current_error)
  Saturation/1 -> Subsystem4/1(V_cmd)
  Rate Transition/1 -> Sum/1
  Subsystem4/1(Im) -> Rate Transition/1
  Subsystem4/2(omega) -> Add/1
  Rate Transition1/1 -> Sum1/1
  Saturation2/1 -> Sum/2

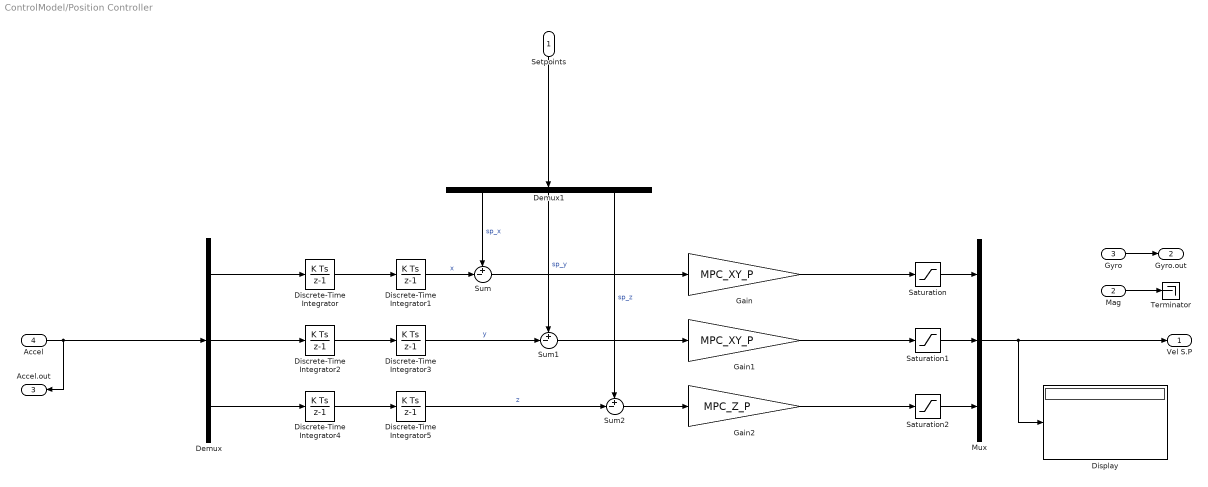
== system ControlModel/Position Controller ==
  Setpoints : Inport
  Mag : Inport  Port=2
  Gyro : Inport  Port=3
  Accel : Inport  Port=4
  Demux : Demux  Outputs=3
  Demux1 : Demux  Outputs=3
  Discrete-Time Integrator : DiscreteIntegrator  SampleTime=Tmech  ICPrevOutput=DiscIntNeverNeededParam  ICPrevScaledInput=DiscIntNeverNeededParam
  Discrete-Time Integrator1 : DiscreteIntegrator  SampleTime=-1  ICPrevOutput=DiscIntNeverNeededParam  ICPrevScaledInput=DiscIntNeverNeededParam
  Discrete-Time Integrator2 : DiscreteIntegrator  SampleTime=Tmech  ICPrevOutput=DiscIntNeverNeededParam  ICPrevScaledInput=DiscIntNeverNeededParam
  Discrete-Time Integrator3 : DiscreteIntegrator  SampleTime=-1  ICPrevOutput=DiscIntNeverNeededParam  ICPrevScaledInput=DiscIntNeverNeededParam
  Discrete-Time Integrator4 : DiscreteIntegrator  SampleTime=Tmech  LimitOutput=on  UpperSaturationLimit=1  ICPrevOutput=DiscIntNeverNeededParam  ICPrevScaledInput=DiscIntNeverNeededParam
  Discrete-Time Integrator5 : DiscreteIntegrator  SampleTime=-1  LimitOutput=on  UpperSaturationLimit=0  ICPrevOutput=DiscIntNeverNeededParam  ICPrevScaledInput=DiscIntNeverNeededParam
  Display : Display
  Gain : Gain  Gain=MPC_XY_P
  Gain1 : Gain  Gain=MPC_XY_P
  Gain2 : Gain  Gain=MPC_Z_P
  Mux : Mux  Inputs=3
  Saturation : Saturate  UpperLimit=MPC_XY_VEL_MAX  LowerLimit=-MPC_XY_VEL_MAX
  Saturation1 : Saturate  UpperLimit=MPC_XY_VEL_MAX  LowerLimit=-MPC_XY_VEL_MAX
  Saturation2 : Saturate  UpperLimit=MPC_Z_VEL_MAX_UP  LowerLimit=MPC_Z_VEL_MAX_DOWN
  Sum : Sum  Inputs=+-|
  Sum1 : Sum  Inputs=+-|
  Sum2 : Sum  Inputs=+-|
  Terminator : Terminator
  Vel S.P : Outport
  Gyro.out : Outport  Port=2
  Accel.out : Outport  Port=3
  wires:
  Mag/1 -> Terminator/1
  Gyro/1 -> Gyro.out/1
  Demux/1 -> Discrete-Time Integrator/1
  Discrete-Time Integrator/1 -> Discrete-Time Integrator1/1
  Demux/2 -> Discrete-Time Integrator2/1
  Demux/3 -> Discrete-Time Integrator4/1
  Discrete-Time Integrator1/1 -> Sum/2  "x"
  Demux1/1 -> Sum/1  "sp_x"
  Discrete-Time Integrator3/1 -> Sum1/2  "y"
  Demux1/2 -> Sum1/1  "sp_y"
  Discrete-Time Integrator5/1 -> Sum2/2  "z"
  Demux1/3 -> Sum2/1  "sp_z"
  Sum/1 -> Gain/1
  Sum1/1 -> Gain1/1
  Sum2/1 -> Gain2/1
  Gain/1 -> Saturation/1
  Gain1/1 -> Saturation1/1
  Gain2/1 -> Saturation2/1
  Saturation2/1 -> Mux/3
  Saturation1/1 -> Mux/2
  Saturation/1 -> Mux/1
  Mux/1 -> Display/1, Vel S.P/1
  Accel/1 -> Demux/1, Accel.out/1
  Discrete-Time Integrator2/1 -> Discrete-Time Integrator3/1
  Discrete-Time Integrator4/1 -> Discrete-Time Integrator5/1
  Setpoints/1 -> Demux1/1

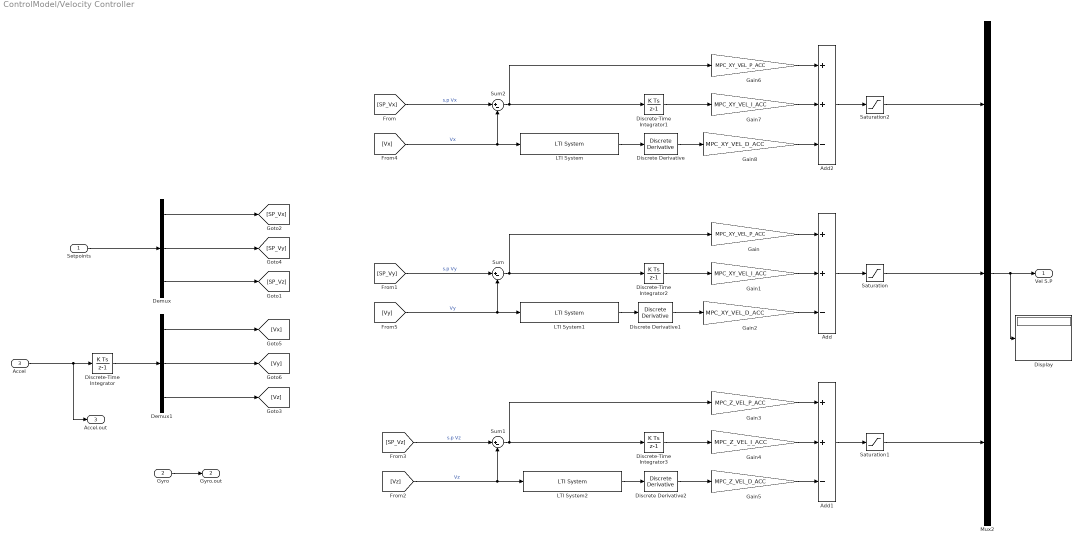
== system ControlModel/Velocity Controller ==
  Setpoints : Inport
  Gyro : Inport  Port=2
  Accel : Inport  Port=3
  Add : Sum  Inputs=++-
  Add1 : Sum  Inputs=++-
  Add2 : Sum  Inputs=++-
  Demux : Demux  Outputs=3
  Demux1 : Demux  Outputs=3
  Discrete Derivative : simulink/Discrete/Discrete Derivative  gainval=1.0  ICPrevScaledInput=0.0  OutMin=[]  OutMax=[]  OutDataType=fixdt(1, 16)  OutScaling=2^-10  DoSatur=off
  Discrete Derivative1 : simulink/Discrete/Discrete Derivative  gainval=1.0  ICPrevScaledInput=0.0  OutMin=[]  OutMax=[]  OutDataType=fixdt(1, 16)  OutScaling=2^-10  DoSatur=off
  Discrete Derivative2 : simulink/Discrete/Discrete Derivative  gainval=1.0  ICPrevScaledInput=0.0  OutMin=[]  OutMax=[]  OutDataType=fixdt(1, 16)  OutScaling=2^-10  DoSatur=off
  Discrete-Time Integrator{,1..3} (4 alike) : DiscreteIntegrator  SampleTime=Tmech  ICPrevOutput=DiscIntNeverNeededParam  ICPrevScaledInput=DiscIntNeverNeededParam
  Display : Display
  Gain : Gain  Gain=MPC_XY_VEL_P_ACC
  Gain1 : Gain  Gain=MPC_XY_VEL_I_ACC
  Gain2 : Gain  Gain=MPC_XY_VEL_D_ACC
  Gain3 : Gain  Gain=MPC_Z_VEL_P_ACC
  Gain4 : Gain  Gain=MPC_Z_VEL_I_ACC
  Gain5 : Gain  Gain=MPC_Z_VEL_D_ACC
  Gain6 : Gain  Gain=MPC_XY_VEL_P_ACC
  Gain7 : Gain  Gain=MPC_XY_VEL_I_ACC
  Gain8 : Gain  Gain=MPC_XY_VEL_D_ACC
  LTI System : cstblocks/LTI System  sys=c2d(tf(1,[MPC_VELD_LP 1]),Tmech)  IC=[]
  LTI System1 : cstblocks/LTI System  sys=c2d(tf(1,[MPC_VELD_LP 1]),Tmech)  IC=[]
  LTI System2 : cstblocks/LTI System  sys=c2d(tf(1,[MPC_VELD_LP 1]),Tmech)  IC=[]
  Mux2 : Mux  Inputs=3
  Saturation : Saturate  UpperLimit=MPC_TILTMAX_AIR  LowerLimit=-MPC_TILTMAX_AIR
  Saturation1 : Saturate  UpperLimit=MPC_THR_MAX  LowerLimit=0
  Saturation2 : Saturate  UpperLimit=MPC_TILTMAX_AIR  LowerLimit=-MPC_TILTMAX_AIR
  Sum : Sum  Inputs=|+-
  Sum1 : Sum  Inputs=|+-
  Sum2 : Sum  Inputs=|+-
  Vel S.P : Outport
  Gyro.out : Outport  Port=2
  Accel.out : Outport  Port=3
  wires:
  Setpoints/1 -> Demux/1
  Demux/3 -> [SP_Vz]
  Gyro/1 -> Gyro.out/1
  Demux1/3 -> [Vz]
  Discrete-Time Integrator/1 -> Demux1/1
  LTI System1/1 -> Discrete Derivative1/1
  Sum/1 -> Discrete-Time Integrator2/1, Gain/1
  Discrete-Time Integrator2/1 -> Gain1/1
  Gain2/1 -> Add/3
  Gain1/1 -> Add/2
  Gain/1 -> Add/1
  Add/1 -> Saturation/1
  Add1/1 -> Saturation1/1
  Gain3/1 -> Add1/1
  Gain4/1 -> Add1/2
  Gain5/1 -> Add1/3
  Discrete-Time Integrator3/1 -> Gain4/1
  Sum1/1 -> Discrete-Time Integrator3/1, Gain3/1
  LTI System2/1 -> Discrete Derivative2/1
  [Vz] -> LTI System2/1, Sum1/2  "Vz"
  [SP_Vz] -> Sum1/1  "s.p Vz"
  Saturation/1 -> Mux2/2
  Mux2/1 -> Display/1, Vel S.P/1
  Add2/1 -> Saturation2/1
  Gain6/1 -> Add2/1
  Gain7/1 -> Add2/2
  Gain8/1 -> Add2/3
  Discrete-Time Integrator1/1 -> Gain7/1
  Sum2/1 -> Discrete-Time Integrator1/1, Gain6/1
  LTI System/1 -> Discrete Derivative/1
  Demux/1 -> [SP_Vx]
  Demux/2 -> [SP_Vy]
  [SP_Vx] -> Sum2/1  "s.p Vx"
  [SP_Vy] -> Sum/1  "s.p Vy"
  Demux1/1 -> [Vx]
  [Vx] -> LTI System/1, Sum2/2  "Vx"
  Demux1/2 -> [Vy]
  [Vy] -> LTI System1/1, Sum/2  "Vy"
  Saturation2/1 -> Mux2/1
  Saturation1/1 -> Mux2/3
  Discrete Derivative/1 -> Gain8/1
  Discrete Derivative1/1 -> Gain2/1
  Discrete Derivative2/1 -> Gain5/1
  Accel/1 -> Discrete-Time Integrator/1, Accel.out/1

== system ControlModel/Attitude Controller/Acceleration to Quaternions1 ==
  acc : Inport
  des_yaw : Inport  Port=2
  Rotation Angles to Quaternions : sharedtransform/Rotation Angles to Quaternions  rotationOrder=ZYX  aMode=aMode
      settings: SourceProductBaseCode=AE,PW,MT,UV,VE,VP
  Terminator : Terminator
  quatVect : MATLAB Function  TreatAsAtomicUnit=on
  Quat : Outport
  wires:
  des_yaw/1 -> quatVect/2(des_yaw)
  acc/1 -> quatVect/1(acc)
  quatVect/2(thrust) -> Terminator/1
  quatVect/1(eulAngles) -> Rotation Angles to Quaternions/1
  Rotation Angles to Quaternions/1 -> Quat/1  "ref_att"

== system ControlModel/Attitude Controller/Norm3 ==
  In1 : Inport
  Math Function : Math  Operator=square  SignedPower=on  SaturateOnIntegerOverflow=on
  Math Function1 : Math  Operator=sqrt  SignedPower=on  SaturateOnIntegerOverflow=on
  Sum of Elements : Sum  Inputs=+
  Out1 : Outport  VectorParamsAs1DForOutWhenUnconnected=off
  wires:
  Sum of Elements/1 -> Math Function1/1
  Math Function/1 -> Sum of Elements/1
  Math Function1/1 -> Out1/1
  In1/1 -> Math Function/1

== system ControlModel/Attitude Controller/Old Calculations ==
  Demux1 : Demux  Commented=on
  Demux2 : Demux  Commented=on
  Euler Angles Transformation : MATLAB Function  Commented=on  TreatAsAtomicUnit=on
  Quaternions Transformation : Subsystem  Commented=on
  Quaternions Transformation - New Version : Subsystem  Commented=on
  Terminator{2..6} (5 alike) : Terminator  Commented=on
  wires:
  Quaternions Transformation - New Version/1(q_e_rp) -> Demux1/1
  Demux2/2 -> Terminator5/1
  Demux2/1 -> Terminator4/1
  Demux1/4 -> Terminator3/1
  Demux1/2 -> ?
  Demux1/3 -> ?
  Demux2/4 -> ?
  Quaternions Transformation - New Version/2(q_e_y) -> Demux2/1
  Demux1/1 -> Terminator2/1
  Demux2/3 -> Terminator6/1

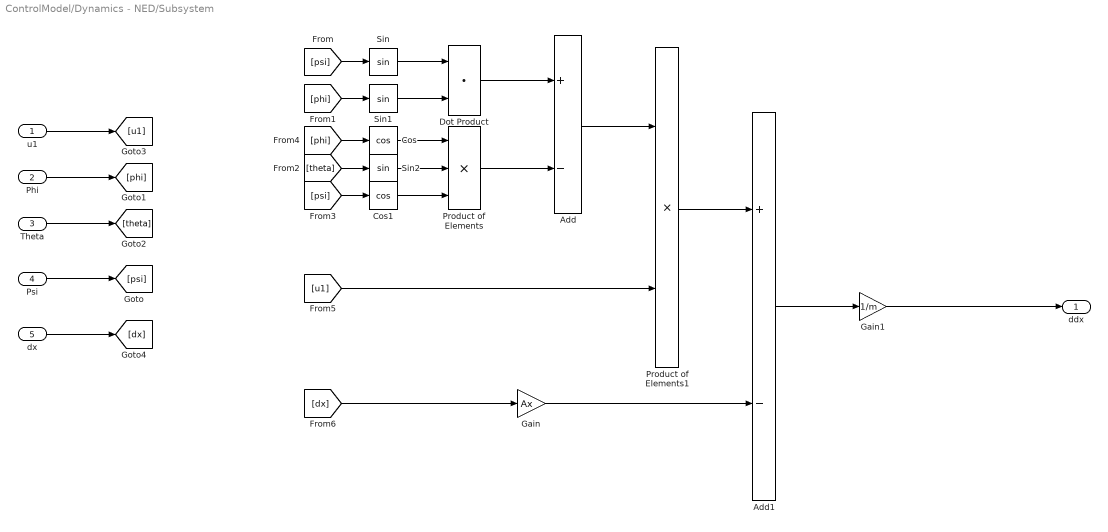
== system ControlModel/Dynamics - NED/Subsystem ==
  u1 : Inport
  Phi : Inport  Port=2
  Theta : Inport  Port=3
  Psi : Inport  Port=4
  dx : Inport  Port=5
  Add : Sum  Inputs=+-
  Add1 : Sum  Inputs=+-
  Cos : Trigonometry  Operator=cos
  Cos1 : Trigonometry  Operator=cos
  Dot Product : DotProduct  InputSameDT=on  OutDataTypeStr=Inherit: Inherit via internal rule
  Gain : Gain  Gain=Ax
  Gain1 : Gain  Gain=1/m
  Product of Elements : Product  Inputs=3
  Product of Elements1 : Product
  Sin : Trigonometry
  Sin1 : Trigonometry
  Sin2 : Trigonometry
  ddx : Outport
  wires:
  Cos/1 -> Product of Elements/1
  [phi] -> Cos/1
  [psi] -> Cos1/1
  Cos1/1 -> Product of Elements/3
  Sin1/1 -> Dot Product/2
  Gain/1 -> Add1/2
  [u1] -> Product of Elements1/2
  Product of Elements/1 -> Add/2
  Product of Elements1/1 -> Add1/1
  Add/1 -> Product of Elements1/1
  [theta] -> Sin2/1
  Sin2/1 -> Product of Elements/2
  [dx] -> Gain/1
  Dot Product/1 -> Add/1
  [psi] -> Sin/1
  Sin/1 -> Dot Product/1
  [phi] -> Sin1/1
  Add1/1 -> Gain1/1
  Psi/1 -> [psi]
  Phi/1 -> [phi]
  Theta/1 -> [theta]
  u1/1 -> [u1]
  dx/1 -> [dx]
  Gain1/1 -> ddx/1

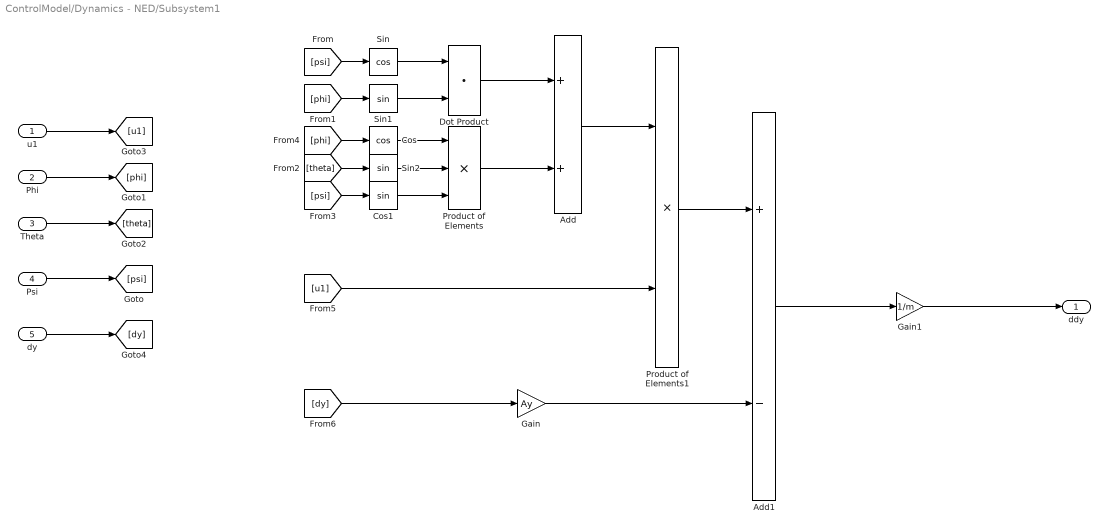
== system ControlModel/Dynamics - NED/Subsystem1 ==
  u1 : Inport
  Phi : Inport  Port=2
  Theta : Inport  Port=3
  Psi : Inport  Port=4
  dy : Inport  Port=5
  Add : Sum
  Add1 : Sum  Inputs=+-
  Cos : Trigonometry  Operator=cos
  Cos1 : Trigonometry
  Dot Product : DotProduct  InputSameDT=on  OutDataTypeStr=Inherit: Inherit via internal rule
  Gain : Gain  Gain=Ay
  Gain1 : Gain  Gain=1/m
  Product of Elements : Product  Inputs=3
  Product of Elements1 : Product
  Sin : Trigonometry  Operator=cos
  Sin1 : Trigonometry
  Sin2 : Trigonometry
  ddy : Outport
  wires:
  dy/1 -> [dy]
  u1/1 -> [u1]
  Theta/1 -> [theta]
  Phi/1 -> [phi]
  Psi/1 -> [psi]
  Add1/1 -> Gain1/1
  [phi] -> Sin1/1
  Sin/1 -> Dot Product/1
  [psi] -> Sin/1
  Dot Product/1 -> Add/1
  [dy] -> Gain/1
  Sin2/1 -> Product of Elements/2
  [theta] -> Sin2/1
  Add/1 -> Product of Elements1/1
  Product of Elements1/1 -> Add1/1
  Product of Elements/1 -> Add/2
  [u1] -> Product of Elements1/2
  Gain/1 -> Add1/2
  Sin1/1 -> Dot Product/2
  Cos1/1 -> Product of Elements/3
  [psi] -> Cos1/1
  [phi] -> Cos/1
  Cos/1 -> Product of Elements/1
  Gain1/1 -> ddy/1

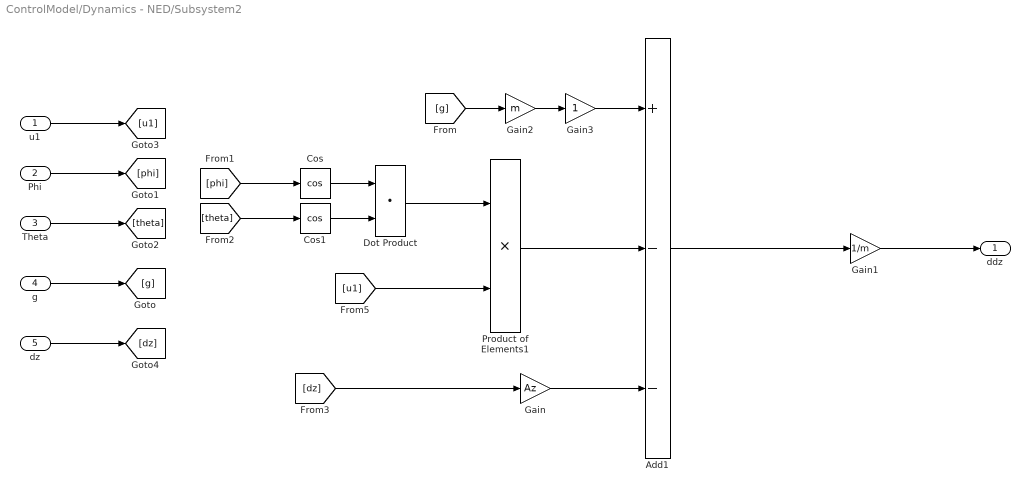
== system ControlModel/Dynamics - NED/Subsystem2 ==
  u1 : Inport
  Phi : Inport  Port=2
  Theta : Inport  Port=3
  g : Inport  Port=4
  dz : Inport  Port=5
  Add1 : Sum  Inputs=+--
  Cos : Trigonometry  Operator=cos
  Cos1 : Trigonometry  Operator=cos
  Dot Product : DotProduct  InputSameDT=on  OutDataTypeStr=Inherit: Inherit via internal rule
  Gain : Gain  Gain=Az
  Gain1 : Gain  Gain=1/m
  Gain2 : Gain  Gain=m
  Gain3 : Gain
      settings: OpenFcn=|
      | a=get_param(gcb,'gain');
      | if a == '1'
      | set_param(gcb,'gain','0','backgroundcolor','red')
      | else
      | set_param(gcb,'gain','1','backgroundcolor','green')
      | end
  Product of Elements1 : Product
  ddz : Outport
  wires:
  Product of Elements1/1 -> Add1/2
  [u1] -> Product of Elements1/2
  Gain2/1 -> Gain3/1
  [dz] -> Gain/1
  Add1/1 -> Gain1/1
  g/1 -> [g]
  Phi/1 -> [phi]
  Theta/1 -> [theta]
  u1/1 -> [u1]
  dz/1 -> [dz]
  Gain/1 -> Add1/3
  [g] -> Gain2/1
  Dot Product/1 -> Product of Elements1/1
  Cos/1 -> Dot Product/1
  [phi] -> Cos/1
  Cos1/1 -> Dot Product/2
  [theta] -> Cos1/1
  Gain3/1 -> Add1/1
  Gain1/1 -> ddz/1
